simulink model "Inductive_Balancing"  (R2024b)
settings: Solver=VariableStepAuto  StartTime=0.0  StopTime=30  RelTol=1e-3
undefined symbols (not defined in the file): Ion, Lithium
libraries: spsIdealSwitchLib x4, spsSeriesRLCBranchLib x4, spsBatteryLib x2, spsDiodeLib x2, spsDCVoltageSourceLib x1, spsGroundLib x1, spsPWMGenerator2LevelLib x1, sps_lib x1
settings Model: Creator=yeswa  LastModifiedBy=yeswa

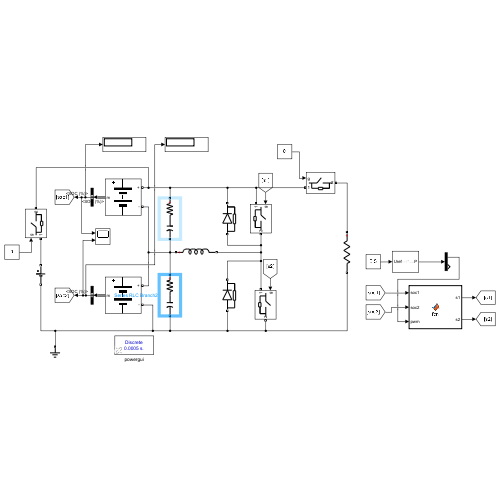
[thumbnail: Simulink's stored preview of the top-level diagram]
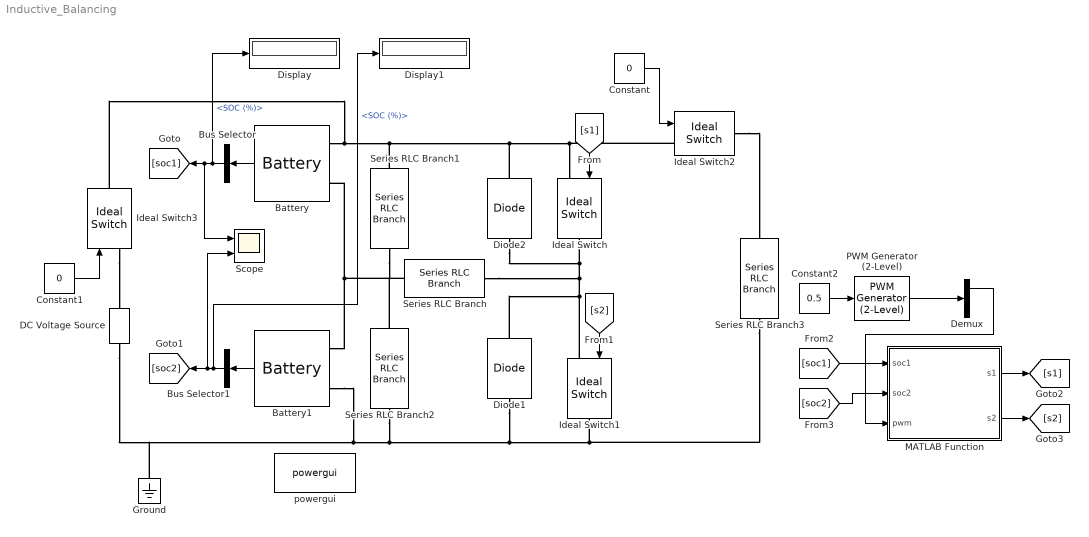
== system Inductive_Balancing ==
  Battery : spsBatteryLib/Battery  BatType=Lithium-Ion  NomV=3.7  NomQ=5.4  SOC=50  Batt_Tr=30  PresetModel=on  MaxQ=5.4  MinV=2.775  FullV=4.3068  Dis_rate=2.3478  R=0.0068519  Normal_OP=4.8835  expZone="[3.9974      0.2653]"
  Battery1 : spsBatteryLib/Battery  BatType=Lithium-Ion  NomV=3.7  NomQ=5.4  SOC=40  Batt_Tr=30  PresetModel=on  MaxQ=5.4  MinV=2.775  FullV=4.3068  Dis_rate=2.3478  R=0.0068519  Normal_OP=4.8835  expZone="[3.9974      0.2653]"
  Bus Selector : BusSelector  OutputSignals=SOC (%)
  Bus Selector1 : BusSelector  OutputSignals=SOC (%)
  Constant : Constant  Value=0
  Constant1 : Constant  Value=0
  Constant2 : Constant  Value=0.5
  DC Voltage Source : spsDCVoltageSourceLib/DC Voltage Source  Amplitude=12  Measurements=None
  Demux : Demux  Outputs=2
  Diode1 : spsDiodeLib/Diode  Ron=0.001  Lon=0  Vf=0.8  IC=0  UseSnubber=0  Rs=500  Cs=250e-9  Measurements=off
  Diode2 : spsDiodeLib/Diode  Ron=0.001  Lon=0  Vf=0.8  IC=0  UseSnubber=0  Rs=500  Cs=250e-9  Measurements=off
  Display : Display
  Display1 : Display
  Ground : spsGroundLib/Ground  LConnTagsString=a
  Ideal Switch{,1..3} (4 alike) : spsIdealSwitchLib/Ideal Switch  Ron=0.001  Lon=0  IC=0  Rs=1e5  Cs=inf  Measurements=off
  MATLAB Function : MATLAB Function  TreatAsAtomicUnit=on
  PWM Generator (2-Level) : spsPWMGenerator2LevelLib/PWM Generator (2-Level)  ModulatorType=Single-phase half-bridge (2 pulses)  ModulatorMode=Unsynchronized  Fc=500  Pc=0  nF=27  MinMax="[ -1  1 ]"  SamplingTechnique=Natural  ModulatingSignals=off  m=0.8  Freq=60  Phase=0  Ts=0  ShowCarrierOutport=off
  Scope : Scope  NumInputPorts=2
  Series RLC Branch : spsSeriesRLCBranchLib/Series RLC Branch  LConnTagsString=__new0  RConnTagsString=__new0  BranchType=L  Resistance=1  Inductance=1e-3  SetiL0=off  InitialCurrent=0  Capacitance=1e-6  Setx0=off  InitialVoltage=0  Measurements=None
  Series RLC Branch1 : spsSeriesRLCBranchLib/Series RLC Branch  LConnTagsString=__new0  RConnTagsString=__new0  BranchType=RC  Resistance=1  Inductance=1e-3  SetiL0=off  InitialCurrent=0  Capacitance=1e-6  Setx0=off  InitialVoltage=0  Measurements=None
  Series RLC Branch2 : spsSeriesRLCBranchLib/Series RLC Branch  LConnTagsString=__new0  RConnTagsString=__new0  BranchType=RC  Resistance=1  Inductance=1e-3  SetiL0=off  InitialCurrent=0  Capacitance=1e-6  Setx0=off  InitialVoltage=0  Measurements=None
  Series RLC Branch3 : spsSeriesRLCBranchLib/Series RLC Branch  LConnTagsString=__new0  RConnTagsString=__new0  BranchType=R  Resistance=1  Inductance=1e-3  SetiL0=off  InitialCurrent=0  Capacitance=1e-6  Setx0=off  InitialVoltage=0  Measurements=None
  powergui : sps_lib/powergui  Priority=1  SimulationMode=Discrete  SampleTime=50e-5  frequency=60  Iterations=50  frequencyindice=0  Pbase=100e6  ErrMax=1e-4  UnitsV=kV  UnitsW=MW  buscounter=0  FunctionMessages=off  echomessages=off  EnableUseOfTLC=off  CurrentSourceSwitches=off  DisableSnubberDevices=off  DisableRonSwitches=off  DisableVfSwitches=off  DisplayEquations=off  AutomaticDiscreteSolvers=off  SolverType=Tustin/Backward Euler (TBE)  Interpol=off  ExternalGateDelay=off  methode=off  Ts=100  x0status=blocks  SPID=on  SwTol=0  HookPort=off  NonlinearTolerance=1e-4  nMaxIteration=100  ContinueOnMaxIteration=off  RestoreLinks=warning  ResistiveCurrentMeasurement=off  Frange=[0:2:500]  Ylog=off  Xlog=on  ShowGrid=off  save=off  variable=ZData  structure=0  ZoomFFT=off  StartTime=0.0  cycles=1  DisplayStyle=1  fundamental=60  FreqAxis=off  MaxFrequency=1000  frequencyindicesteady=1  RmsSteady=1  display=off
  wires:
  [s1] -> Ideal Switch/1
  [s2] -> Ideal Switch1/1
  Battery/1 -> Bus Selector/1
  Bus Selector/1 -> Display/1, Scope/1, [soc1]  "<SOC (%)>"
  Battery1/1 -> Bus Selector1/1
  Bus Selector1/1 -> Display1/1, Scope/2, [soc2]  "<SOC (%)>"
  Constant/1 -> Ideal Switch2/1
  Constant1/1 -> Ideal Switch3/1
  Constant2/1 -> PWM Generator (2-Level)/1
  PWM Generator (2-Level)/1 -> Demux/1
  [soc1] -> MATLAB Function/1(soc1)
  [soc2] -> MATLAB Function/2(soc2)
  Demux/1 -> MATLAB Function/3(pwm)
  MATLAB Function/1(s1) -> [s1]
  MATLAB Function/2(s2) -> [s2]
  connections:
  Battery/LConn1 -- Ideal Switch3/RConn1 -- Ideal Switch/LConn1 -- Ideal Switch2/LConn1 -- Diode2/RConn1 -- Series RLC Branch1/LConn1
  Battery1/LConn1 -- Series RLC Branch2/LConn1 -- Series RLC Branch/LConn1 -- Series RLC Branch1/RConn1 -- Battery/LConn2
  Battery1/LConn2 -- Ground/LConn1 -- DC Voltage Source/LConn1 -- Diode1/LConn1 -- Series RLC Branch3/RConn1 -- Ideal Switch1/RConn1 -- Series RLC Branch2/RConn1
  Ideal Switch1/LConn1 -- Diode1/RConn1 -- Diode2/LConn1 -- Ideal Switch/RConn1 -- Series RLC Branch/RConn1
  Ideal Switch2/RConn1 -- Series RLC Branch3/LConn1
  Ideal Switch3/LConn1 -- DC Voltage Source/RConn1

== matlab function Inductive_Balancing/MATLAB Function ==
  data: soc1 input; s1 output; soc2 input; s2 output; pwm input
function [s1,s2] = fcn(soc1,soc2,pwm)
    % Use a persistent counter
    persistent stepCount
    if isempty(stepCount)
        stepCount = 0;
    end

    % Increment counter
    stepCount = stepCount + 1;

    % Core logic
    if soc1 > soc2
        s1 = pwm;
        s2 = 0;
    elseif soc2 > soc1
        s2 = pwm;
        s1 = 0;
    else
        s1 = 0;
        s2 = 0;
    end

    % Debug print for first 100 steps (cast to int32 for %d)
    if stepCount <= 200
        fprintf('Step %d: soc1=%.2f, soc2=%.2f, pwm=%.2f => s1=%.2f, s2=%.2f\n', ...
            int32(stepCount), soc1, soc2, pwm, s1, s2);
    end
end
